simulink model "motortorque_ripple"  (R2013a)
settings: Solver=ode4  StartTime=0.0  StopTime=10  FixedStep=1e-5  RelTol=1e-3
values from neighbouring files (symbols this model uses):
  phase = 3    [mmf_dist.m]    (also in mmf_dist_diffmc.m; mmf_dist_grouped.m; mmf_dist_otherphase.m)
undefined symbols (not defined in the file or in its folder): ma, Ts, wout
libraries: powerlib x13, AC6DriveInternalModels x7, electricdrivelib x3, DriveInternalModels x2, powerlib_meascontrol x1
settings Model: Creator=ugurm  LastModifiedBy=ugurm

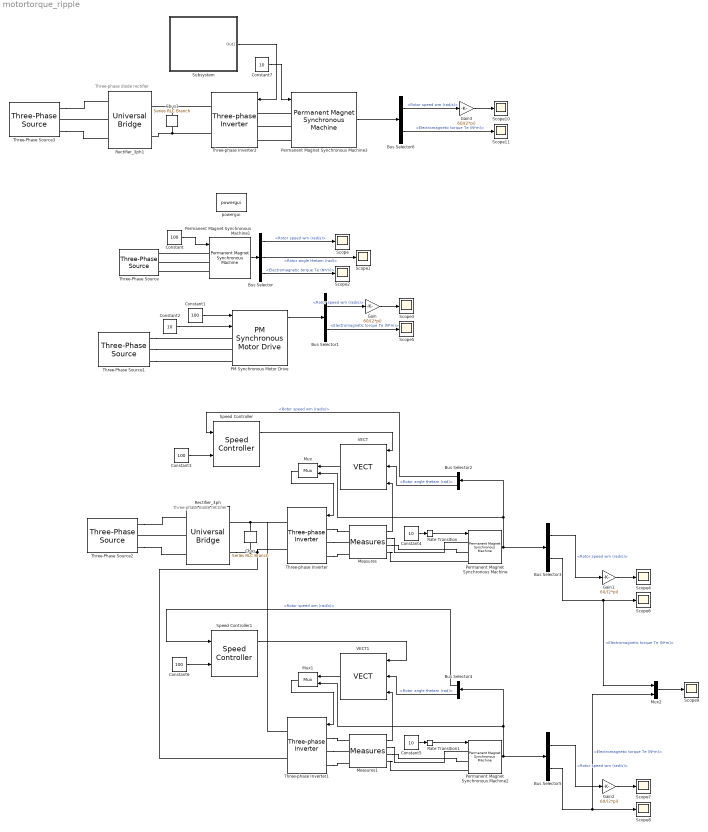
== system motortorque_ripple ==
  note: Three-phase
      | diode rectifier
  note: Three-phase
      | diode rectifier
  Bus Selector : BusSelector  OutputSignals=Rotor speed wm (rad/s),Rotor angle thetam (rad),Electromagnetic torque Te (N*m)
  Bus Selector{1,3,5..6} (4 alike) : BusSelector  OutputSignals=Rotor speed wm (rad/s),Electromagnetic torque Te (N*m)
  Bus Selector2 : BusSelector  OutputSignals=Rotor speed wm (rad/s),Rotor angle thetam (rad)
  Bus Selector4 : BusSelector  OutputSignals=Rotor speed wm (rad/s),Rotor angle thetam (rad)
  Cbus : powerlib/Elements/Series RLC Branch  LConnTagsString=__new0  RConnTagsString=__new0  BranchType=C  Resistance=[]  Inductance=[]  SetiL0=off  InitialCurrent=0  Capacitance=2e-3  Setx0=off  InitialVoltage=0  Measurements=None
  Cbus1 : powerlib/Elements/Series RLC Branch  LConnTagsString=__new0  RConnTagsString=__new0  BranchType=C  Resistance=[]  Inductance=[]  SetiL0=off  InitialCurrent=0  Capacitance=2e-3  Setx0=off  InitialVoltage=0  Measurements=None
  Constant{,1,3,6} (4 alike) : Constant  Value=100
  Constant{2,4..5,7} (4 alike) : Constant  Value=10
  Gain{,1..3} (4 alike) : Gain  Gain=60/(2*pi)
  Measures : electricdrivelib/AC drives/PM Synchronous Motor Drive/Measures
  Measures1 : electricdrivelib/AC drives/PM Synchronous Motor Drive/Measures
  Mux : AC6DriveInternalModels/Mux
  Mux1 : AC6DriveInternalModels/Mux
  Mux2 : Mux  Inputs=2
  PM Synchronous Motor Drive : electricdrivelib/AC drives/PM Synchronous Motor Drive  showMaskWarnings=on  AverageValue=off  MechanicalLoad=Speed w  driveType=AC6
  Permanent Magnet Synchronous Machine : powerlib/Machines/Permanent Magnet Synchronous Machine  NbPhases=3  FluxDistribution=Sinusoidal  RotorType=Salient-pole  MechanicalLoad=Speed w  PresetModel=No  ShowDetailedParameters=on  Resistance=0.2  Inductance=0  dqInductances=[8.5e-3,8.5e-3]  La=0.000835  MachineConstant=Flux linkage established by magnets (V.s)  Flux=0.175  VoltageCst=126.966  TorqueCst=1.05  Flat=0  Mechanical=[0.089,0.005,4]  PolePairs=4  InitialConditions=[0,0, 0,0]  InitialConditions5ph=[0 0 0 0 0 0]  TsPowergui=0  TsBlock=-1  RefAngle=90 degrees behind phase A axis (modified Park)
      settings: AttributesFormatString=\n
  Permanent Magnet Synchronous Machine1 : powerlib/Machines/Permanent Magnet Synchronous Machine  NbPhases=3  FluxDistribution=Sinusoidal  RotorType=Round  MechanicalLoad=Torque Tm  PresetModel="09:  7.14 Nm 560 Vdc 5000 RPM - 8.3 Nm"  ShowDetailedParameters=on  Resistance=0.18  Inductance=8.5e-3  dqInductances=[8.5e-3,8.5e-3]  La=0.000835  MachineConstant=Flux linkage established by magnets (V.s)  Flux=0.07145  VoltageCst=51.8384  TorqueCst=0.4287  Flat=120  Mechanical=[0.00048 0.0001619 4 0]  PolePairs=4  InitialConditions=[0,0, 0,0]  InitialConditions5ph=[0 0 0 0 0 0]  TsPowergui=0  TsBlock=-1  RefAngle=90 degrees behind phase A axis (modified Park)
  Permanent Magnet Synchronous Machine2 : powerlib/Machines/Permanent Magnet Synchronous Machine  NbPhases=3  FluxDistribution=Sinusoidal  RotorType=Salient-pole  MechanicalLoad=Speed w  PresetModel=No  ShowDetailedParameters=on  Resistance=0.2  Inductance=0  dqInductances=[8.5e-3,8.5e-3]  La=0.000835  MachineConstant=Flux linkage established by magnets (V.s)  Flux=0.175  VoltageCst=126.966  TorqueCst=1.05  Flat=0  Mechanical=[0.089,0.005,4]  PolePairs=4  InitialConditions=[0,0, 0,0]  InitialConditions5ph=[0 0 0 0 0 0]  TsPowergui=0  TsBlock=-1  RefAngle=90 degrees behind phase A axis (modified Park)
      settings: AttributesFormatString=\n
  Permanent Magnet Synchronous Machine3 : powerlib/Machines/Permanent Magnet Synchronous Machine  NbPhases=3  FluxDistribution=Sinusoidal  RotorType=Salient-pole  MechanicalLoad=Speed w  PresetModel=No  ShowDetailedParameters=on  Resistance=0.2  Inductance=0  dqInductances=[8.5e-3,8.5e-3]  La=0.000835  MachineConstant=Flux linkage established by magnets (V.s)  Flux=0.175  VoltageCst=126.966  TorqueCst=1.05  Flat=0  Mechanical=[0.089,0.005,4]  PolePairs=4  InitialConditions=[0,0, 0,0]  InitialConditions5ph=[0 0 0 0 0 0]  TsPowergui=0  TsBlock=-1  RefAngle=90 degrees behind phase A axis (modified Park)
      settings: AttributesFormatString=\n
  Rate Transition : RateTransition  OutPortSampleTime=Ts
  Rate Transition1 : RateTransition  OutPortSampleTime=Ts
  Rectifier_3ph : powerlib/Power Electronics/Universal Bridge  Arms=3  SnubberResistance=10e3  SnubberCapacitance=20e-9  Device=Diodes  Ron=1e-3  Lon=0  ForwardVoltages="[  0,  0  ]"  ForwardVoltage=1.3  GTOparameters=[ 10e-6, 20e-6 ]  IGBTparameters=[ 1e-6 , 2e-6 ]  Measurements=All voltages and currents  Measurements_2=None  converterType=Rectifier
  Rectifier_3ph1 : powerlib/Power Electronics/Universal Bridge  Arms=3  SnubberResistance=10e3  SnubberCapacitance=20e-9  Device=Diodes  Ron=1e-3  Lon=0  ForwardVoltages="[  0,  0  ]"  ForwardVoltage=1.3  GTOparameters=[ 10e-6, 20e-6 ]  IGBTparameters=[ 1e-6 , 2e-6 ]  Measurements=All voltages and currents  Measurements_2=None  converterType=Rectifier
  Scope{,1..11} (12 alike) : Scope
      Scope10 settings: YMin=90.7184  YMax=100.268  SaveName=ScopeData10
      Scope11 settings: YMin=-30  YMax=10  SaveName=ScopeData11
      Scope2 settings: SaveName=ScopeData2
      Scope3 settings: YMin=95.493  YMax=95.493  SaveName=ScopeData3
      Scope4 settings: YMin=90.7184  YMax=100.268  SaveName=ScopeData4
      Scope5 settings: YMin=-20  YMax=20  SaveName=ScopeData5
      Scope6 settings: YMin=-20  YMax=20  SaveName=ScopeData6
      Scope7 settings: YMin=95.493  YMax=95.493  SaveName=ScopeData7
      Scope8 settings: YMin=-20  YMax=20  SaveName=ScopeData8
      Scope9 settings: YMin=15.5  YMax=19.75  SaveName=ScopeData9
  Speed Controller : DriveInternalModels/AC drives/Speed Controller AC67/Speed Controller  SwK=Speed regulation  ramp=[-1000,1000]  kp=5  ki=100  fc=100  ctrl_sat=[-17.8,17.8]  Tsc=7*20e-6
  Speed Controller1 : DriveInternalModels/AC drives/Speed Controller AC67/Speed Controller  SwK=Speed regulation  ramp=[-1000,1000]  kp=5  ki=100  fc=100  ctrl_sat=[-17.8,17.8]  Tsc=7*20e-6
  Subsystem : Subsystem
  Three-Phase Source{,1..3} (4 alike) : powerlib/Electrical Sources/Three-Phase Source  Voltage=400  PhaseAngle=0  Frequency=50  InternalConnection=Yg  SpecifyImpedance=off  Resistance=0  Inductance=0  ShortCircuitLevel=100e6  BaseVoltage=400  XRratio=7  BusType=swing  Pref=0  Qref=0  Qmin=-inf  Qmax=inf
  Three-phase Inverter : AC6DriveInternalModels/Three-phase Inverter  Arms=3  SnubberResistance=5000  SnubberCapacitance=inf  Device=IGBT / Diodes  Ron=1e-3  Lon=0  ForwardVoltages=[0.8,0.8]  ForwardVoltage=0  GTOparameters=[0,0]  IGBTParameters=[1e-6,2e-6]  Measurements=All voltages and currents  converterType=Inverter  SourceFrequency=60  dqInductances=[8.5e-3,8.5e-3]  Flux=0.175  Resistance=0.2  p=4
  Three-phase Inverter1 : AC6DriveInternalModels/Three-phase Inverter  Arms=3  SnubberResistance=5000  SnubberCapacitance=inf  Device=IGBT / Diodes  Ron=1e-3  Lon=0  ForwardVoltages=[0.8,0.8]  ForwardVoltage=0  GTOparameters=[0,0]  IGBTParameters=[1e-6,2e-6]  Measurements=All voltages and currents  converterType=Inverter  SourceFrequency=60  dqInductances=[8.5e-3,8.5e-3]  Flux=0.175  Resistance=0.2  p=4
  Three-phase Inverter2 : AC6DriveInternalModels/Three-phase Inverter  Arms=3  SnubberResistance=5000  SnubberCapacitance=inf  Device=IGBT / Diodes  Ron=1e-3  Lon=0  ForwardVoltages=[0.8,0.8]  ForwardVoltage=0  GTOparameters=[0,0]  IGBTParameters=[1e-6,2e-6]  Measurements=All voltages and currents  converterType=Inverter  SourceFrequency=60  dqInductances=[8.5e-3,8.5e-3]  Flux=0.175  Resistance=0.2  p=4
  VECT : AC6DriveInternalModels/VECT  nb_p=4  lambda=0.175  freq_max=20e3  Ts_vect=20e-6  h=0.1
  VECT1 : AC6DriveInternalModels/VECT  nb_p=4  lambda=0.175  freq_max=20e3  Ts_vect=20e-6  h=0.1
  powergui : powerlib/powergui  Priority=1  SimulationMode=Discrete  SolverType=Tustin  SampleTime=1e-5  frequency=60  SPID=off  DisableSnubberDevices=off  DisableRonSwitches=off  DisableVfSwitches=off  SwTol=0  Interpol=off  DisplayEquations=off  frequencyindice=0  Pbase=100e6  ErrMax=1e-4  Iterations=50  UnitsV=kV  UnitsW=MW  FunctionMessages=off  echomessages=off  HookPort=off  EnableUseOfTLC=off  x0status=blocks  RestoreLinks=warning  ResistiveCurrentMeasurement=off  Frange=[0:2:500]  Ylog=off  Xlog=on  ShowGrid=off  save=off  variable=ZData  structure=idc6  ZoomFFT=off  StartTime=0.01  cycles=2  DisplayStyle=6  fundamental=50  FreqAxis=off  MaxFrequency=1000  frequencyindicesteady=1  RmsSteady=1  display=off  Ts=0  methode=off
  wires:
  Permanent Magnet Synchronous Machine1/1 -> Bus Selector/1
  Bus Selector/1 -> Scope/1  "<Rotor speed wm (rad/s)>"
  Bus Selector/2 -> Scope1/1  "<Rotor angle thetam (rad)>"
  Bus Selector/3 -> Scope2/1  "<Electromagnetic torque Te (N*m)>"
  Constant/1 -> Permanent Magnet Synchronous Machine1/1
  Constant1/1 -> PM Synchronous Motor Drive/1
  Constant2/1 -> PM Synchronous Motor Drive/2
  PM Synchronous Motor Drive/1 -> Bus Selector1/1
  Bus Selector1/1 -> Gain/1  "<Rotor speed wm (rad/s)>"
  Bus Selector1/2 -> Scope5/1  "<Electromagnetic torque Te (N*m)>"
  Gain/1 -> Scope3/1
  Rate Transition/1 -> Permanent Magnet Synchronous Machine/1
  Constant4/1 -> Rate Transition/1
  Constant3/1 -> Speed Controller/2
  Measures/1 -> VECT/3
  Speed Controller/1 -> VECT/1
  VECT/1 -> Mux/1
  Mux/1 -> Three-phase Inverter/1
  Bus Selector2/1 -> Speed Controller/1  "<Rotor speed wm (rad/s)>"
  Bus Selector2/2 -> VECT/2  "<Rotor angle thetam (rad)>"
  Permanent Magnet Synchronous Machine/1 -> Bus Selector3/1, Mux/2, Bus Selector2/1
  Bus Selector3/1 -> Gain1/1  "<Rotor speed wm (rad/s)>"
  Bus Selector3/2 -> Mux2/1, Scope6/1  "<Electromagnetic torque Te (N*m)>"
  Gain1/1 -> Scope4/1
  Rate Transition1/1 -> Permanent Magnet Synchronous Machine2/1
  Constant5/1 -> Rate Transition1/1
  Measures1/1 -> VECT1/3
  Speed Controller1/1 -> VECT1/1
  VECT1/1 -> Mux1/1
  Mux1/1 -> Three-phase Inverter1/1
  Bus Selector4/1 -> Speed Controller1/1  "<Rotor speed wm (rad/s)>"
  Bus Selector4/2 -> VECT1/2  "<Rotor angle thetam (rad)>"
  Permanent Magnet Synchronous Machine2/1 -> Bus Selector5/1, Mux1/2, Bus Selector4/1
  Bus Selector5/1 -> Gain2/1  "<Rotor speed wm (rad/s)>"
  Bus Selector5/2 -> Mux2/2, Scope8/1  "<Electromagnetic torque Te (N*m)>"
  Gain2/1 -> Scope7/1
  Constant6/1 -> Speed Controller1/2
  Mux2/1 -> Scope9/1
  Constant7/1 -> Permanent Magnet Synchronous Machine3/1
  Permanent Magnet Synchronous Machine3/1 -> Bus Selector6/1
  Bus Selector6/1 -> Gain3/1  "<Rotor speed wm (rad/s)>"
  Bus Selector6/2 -> Scope11/1  "<Electromagnetic torque Te (N*m)>"
  Gain3/1 -> Scope10/1
  Subsystem/1(Out1) -> Three-phase Inverter2/1
  connections:
  Permanent Magnet Synchronous Machine1/LConn1 -- Three-Phase Source/RConn1
  Permanent Magnet Synchronous Machine1/LConn2 -- Three-Phase Source/RConn2
  Permanent Magnet Synchronous Machine1/LConn3 -- Three-Phase Source/RConn3
  Three-Phase Source1/RConn3 -- PM Synchronous Motor Drive/LConn3
  Three-Phase Source1/RConn2 -- PM Synchronous Motor Drive/LConn2
  Three-Phase Source1/RConn1 -- PM Synchronous Motor Drive/LConn1
  Cbus/LConn1 -- Three-phase Inverter1/RConn1 -- Three-phase Inverter/RConn1 -- Rectifier_3ph/RConn1
  Measures/RConn3 -- Permanent Magnet Synchronous Machine/LConn3
  Measures/RConn2 -- Permanent Magnet Synchronous Machine/LConn2
  Measures/RConn1 -- Permanent Magnet Synchronous Machine/LConn1
  Three-phase Inverter/LConn1 -- Measures/LConn1
  Rectifier_3ph/LConn2 -- Three-Phase Source2/RConn2
  Three-phase Inverter/LConn3 -- Measures/LConn3
  Three-Phase Source2/RConn3 -- Rectifier_3ph/LConn3
  Three-Phase Source2/RConn1 -- Rectifier_3ph/LConn1
  Three-phase Inverter/LConn2 -- Measures/LConn2
  Rectifier_3ph/RConn2 -- Cbus/RConn1 -- Three-phase Inverter1/RConn2 -- Three-phase Inverter/RConn2
  Measures1/RConn1 -- Permanent Magnet Synchronous Machine2/LConn1
  Measures1/RConn3 -- Permanent Magnet Synchronous Machine2/LConn3
  Three-phase Inverter1/LConn1 -- Measures1/LConn1
  Measures1/RConn2 -- Permanent Magnet Synchronous Machine2/LConn2
  Three-phase Inverter1/LConn3 -- Measures1/LConn3
  Three-phase Inverter1/LConn2 -- Measures1/LConn2
  Permanent Magnet Synchronous Machine3/LConn1 -- Three-phase Inverter2/LConn1
  Permanent Magnet Synchronous Machine3/LConn2 -- Three-phase Inverter2/LConn2
  Permanent Magnet Synchronous Machine3/LConn3 -- Three-phase Inverter2/LConn3
  Cbus1/LConn1 -- Three-phase Inverter2/RConn1 -- Rectifier_3ph1/RConn1
  Rectifier_3ph1/RConn2 -- Three-phase Inverter2/RConn2 -- Cbus1/RConn1
  Three-Phase Source3/RConn3 -- Rectifier_3ph1/LConn3
  Rectifier_3ph1/LConn2 -- Three-Phase Source3/RConn2
  Three-Phase Source3/RConn1 -- Rectifier_3ph1/LConn1

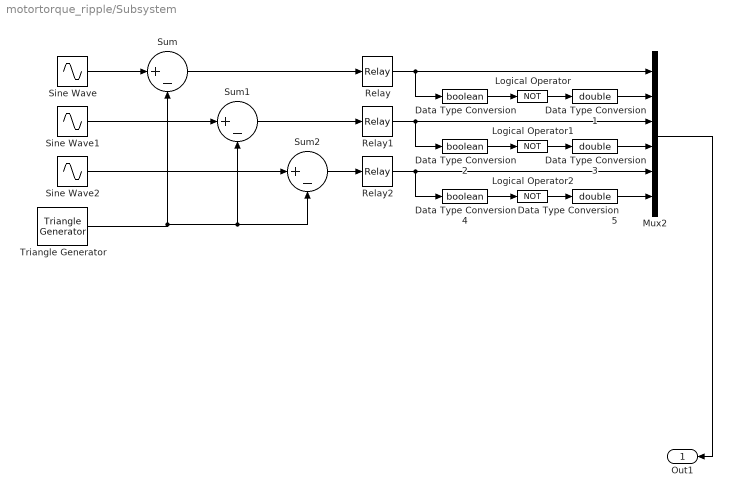
== system motortorque_ripple/Subsystem ==
  Data Type Conversion : DataTypeConversion  OutDataTypeStr=boolean
  Data Type Conversion1 : DataTypeConversion  OutDataTypeStr=double
  Data Type Conversion2 : DataTypeConversion  OutDataTypeStr=boolean
  Data Type Conversion3 : DataTypeConversion  OutDataTypeStr=double
  Data Type Conversion4 : DataTypeConversion  OutDataTypeStr=boolean
  Data Type Conversion5 : DataTypeConversion  OutDataTypeStr=double
  Logical Operator : Logic  Operator=NOT  AllPortsSameDT=off  OutDataTypeStr=boolean
  Logical Operator1 : Logic  Operator=NOT  AllPortsSameDT=off  OutDataTypeStr=boolean
  Logical Operator2 : Logic  Operator=NOT  AllPortsSameDT=off  OutDataTypeStr=boolean
  Mux2 : Mux  Inputs=6
  Relay : Relay
  Relay1 : Relay
  Relay2 : Relay
  Sine Wave : Sin  Amplitude=ma  Frequency=wout  SampleTime=0
  Sine Wave1 : Sin  Amplitude=ma  Frequency=wout  Phase=-2*pi/3  SampleTime=0
  Sine Wave2 : Sin  Amplitude=ma  Frequency=wout  Phase=2*pi/3  SampleTime=0
  Sum : Sum  Inputs=|+-
  Sum1 : Sum  Inputs=|+-
  Sum2 : Sum  Inputs=|+-
  Triangle Generator : powerlib_meascontrol/Pulse & Signal Generators/Triangle Generator  Freq=fsw  Phase=0  Ts=Ts
  Out1 : Outport
  wires:
  Logical Operator1/1 -> Data Type Conversion3/1
  Sum/1 -> Relay/1
  Triangle Generator/1 -> Sum1/2, Sum2/2, Sum/2
  Logical Operator/1 -> Data Type Conversion1/1
  Relay1/1 -> Data Type Conversion2/1, Mux2/3
  Logical Operator2/1 -> Data Type Conversion5/1
  Data Type Conversion4/1 -> Logical Operator2/1
  Data Type Conversion2/1 -> Logical Operator1/1
  Data Type Conversion5/1 -> Mux2/6
  Sine Wave2/1 -> Sum2/1
  Data Type Conversion3/1 -> Mux2/4
  Sum1/1 -> Relay1/1
  Relay2/1 -> Data Type Conversion4/1, Mux2/5
  Relay/1 -> Data Type Conversion/1, Mux2/1
  Mux2/1 -> Out1/1
  Data Type Conversion1/1 -> Mux2/2
  Sine Wave/1 -> Sum/1
  Sine Wave1/1 -> Sum1/1
  Data Type Conversion/1 -> Logical Operator/1
  Sum2/1 -> Relay2/1
